simulink model "Constants"  (R2021a)
settings: Solver=FixedStepAuto  StartTime=0.0  StopTime=50  FixedStep=1e-3  RelTol=1e-3  EnableMultiTasking=on
undefined symbols (not defined in the file): D0, D1, D10, D11, D12, D13, D2, D3, D4, D5, D6, D7, D8, D9, magnitude, PTA0, PTA1, PTA2, PTB23, PTB9, PTC16, PTC17, PTC2, PTC3, PTC4, PTD0, PTD1, PTD2, PTD3
libraries: frdmk64flib x19, dspstat3 x1
settings Model: SimulationMode=external  PacingRate=0.250000  ExtModeTrigDuration=5  Creator=Arun Mistry  LastModifiedBy=Arun Mistry
settings OptimizationCC: EnhancedBackFolding=on  PassReuseOutputArgsAs=Individual arguments  ZeroExternalMemoryAtStartup=off  ZeroInternalMemoryAtStartup=off  MaxStackSize=64  OptimizeBlockOrder=speed  DifferentSizesBufferReuse=on  OptimizationCustomize=off  EfficientTunableParamExpr=on
settings DebuggingCC: ParameterTunabilityLossMsg=error
settings HardwareCC: ProdBitPerPointer=32  ProdBitPerSizeT=32  ProdBitPerPtrDiffT=32  ProdLargestAtomicInteger=Long  ProdLargestAtomicFloat=Double  ProdWordSize=32  ProdHWDeviceType=ARM Compatible->ARM Cortex
settings SFSimCC: MATLABDynamicMemAlloc=off
settings RTWCC: SystemTargetFile=ert.tlc  HardwareBoard=NXP FRDM-K64F  TLCOptions="-aInlineSetEventsForThisBaseRateFcn=TLC_FALSE -aSuppressMultiTaskScheduler=TLC_FALSE  -aRateBasedStepFcn=0"  TemplateMakefile=ert_default_tmf  Toolchain=GNU Tools for ARM Embedded Processors
settings CodeAppCC: ForceParamTrailComments=on  IgnoreCustomStorageClasses=off  OperatorAnnotations=on  SimulinkDataObjDesc=on  SFDataObjDesc=on  InsertBlockDesc=on
settings ERTTargetCC: ExtModeTransport=4  ExtModeMexFile=sendToCommService

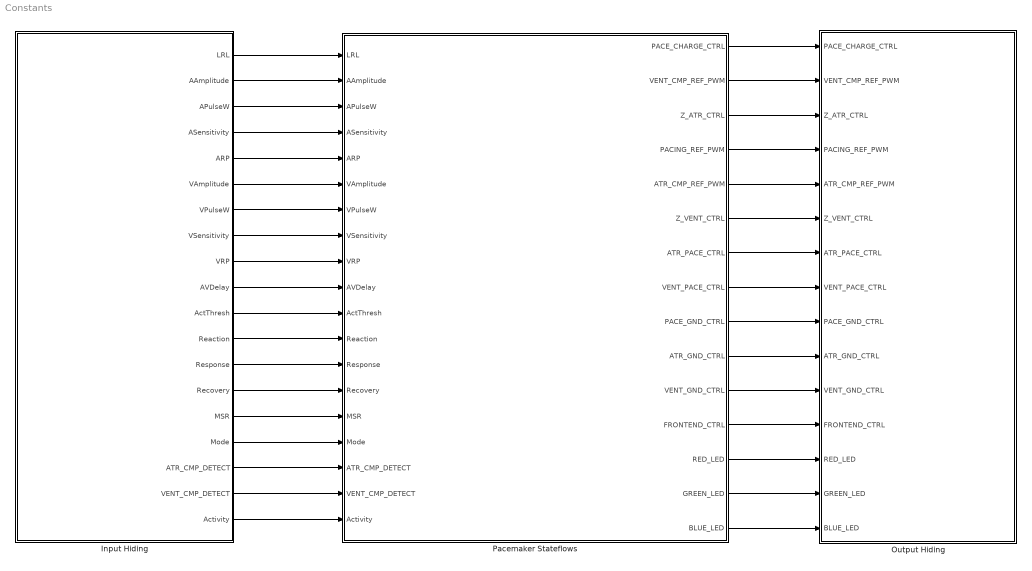
== system Constants ==
  Input Hiding : Subsystem
  Output Hiding : Subsystem
  Pacemaker Stateflows : Stateflow chart  TreatAsAtomicUnit=on
      settings: PortSchema="{\"entries\":[{\"content\":{\"sides\":[{\"content\":{\"connectorIds\":[\"In1\",\"In2\",\"In3\",\"In4\",\"In5\",\"In6\",\"In7\",\"In8\",\"In9\",\"In17\",\"In11\",\"In10\",\"In12\",\"In14\",\"In19\",\"In13\",\"In15\",\"In16\",\"In18\"]},\"type\":\"ConnectorPlacement.EquallySpacedRectSide\",\"uuid\":\"6f24296b-9994-4871-8227-e053a3629335\"},{\"content\":{\"connectorIds\":[\"Out1\",\"Out2\",\"Out3\",\"Out4\",\"Out5\",\"Out6\",\"Out7\",\"Out8\",\"Out9\",\"Out10\",\"Out11\",\"Out12\",\"Out13\",\"Out14\",\"Out15\"],\"side\":\"RIGHT\"},\"type\":\"ConnectorPlacement.EquallySpacedRectSide\",\"uuid\":\"36cf1f29-c3ea-48aa-b003-da737efff16a\"},{\"content\":{\"connectorIds\":[],\"side\":\"TOP\"},\"type\":\"ConnectorPlacement.EquallySpacedRectSide\",\"uuid\":\"8330eb51-0bc3-4d96-96ed-331fbb159cdb\"}]},\"type\":\"ConnectorPlacement.EquallySpacedConnector\",\"uuid\":\"1e79ed8a-065e-4a3c-97dd-23eb49490e0b\"}],\"packageUris\":[\"http://schema.mathworks.com/mf0/Connector/R2020b\"],\"version\":\"1.0\"}"
  wires:
  Pacemaker Stateflows/1(PACE_CHARGE_CTRL) -> Output Hiding/1(PACE_CHARGE_CTRL)
  Input Hiding/17(ATR_CMP_DETECT) -> Pacemaker Stateflows/15(ATR_CMP_DETECT)
  Input Hiding/7(VPulseW) -> Pacemaker Stateflows/7(VPulseW)
  Input Hiding/18(VENT_CMP_DETECT) -> Pacemaker Stateflows/16(VENT_CMP_DETECT)
  Pacemaker Stateflows/3(Z_ATR_CTRL) -> Output Hiding/3(Z_ATR_CTRL)
  Input Hiding/3(APulseW) -> Pacemaker Stateflows/3(APulseW)
  Pacemaker Stateflows/7(ATR_PACE_CTRL) -> Output Hiding/7(ATR_PACE_CTRL)
  Pacemaker Stateflows/10(ATR_GND_CTRL) -> Output Hiding/10(ATR_GND_CTRL)
  Input Hiding/16(Mode) -> Pacemaker Stateflows/13(Mode)
  Input Hiding/2(AAmplitude) -> Pacemaker Stateflows/2(AAmplitude)
  Input Hiding/6(VAmplitude) -> Pacemaker Stateflows/6(VAmplitude)
  Pacemaker Stateflows/6(Z_VENT_CTRL) -> Output Hiding/6(Z_VENT_CTRL)
  Pacemaker Stateflows/4(PACING_REF_PWM) -> Output Hiding/4(PACING_REF_PWM)
  Pacemaker Stateflows/11(VENT_GND_CTRL) -> Output Hiding/11(VENT_GND_CTRL)
  Pacemaker Stateflows/9(PACE_GND_CTRL) -> Output Hiding/9(PACE_GND_CTRL)
  Pacemaker Stateflows/8(VENT_PACE_CTRL) -> Output Hiding/8(VENT_PACE_CTRL)
  Input Hiding/1(LRL) -> Pacemaker Stateflows/1(LRL)
  Pacemaker Stateflows/15(BLUE_LED) -> Output Hiding/15(BLUE_LED)
  Input Hiding/4(ASensitivity) -> Pacemaker Stateflows/4(ASensitivity)
  Pacemaker Stateflows/12(FRONTEND_CTRL) -> Output Hiding/12(FRONTEND_CTRL)
  Input Hiding/9(VRP) -> Pacemaker Stateflows/9(VRP)
  Input Hiding/8(VSensitivity) -> Pacemaker Stateflows/8(VSensitivity)
  Input Hiding/5(ARP) -> Pacemaker Stateflows/5(ARP)
  Pacemaker Stateflows/14(GREEN_LED) -> Output Hiding/14(GREEN_LED)
  Pacemaker Stateflows/13(RED_LED) -> Output Hiding/13(RED_LED)
  Pacemaker Stateflows/5(ATR_CMP_REF_PWM) -> Output Hiding/5(ATR_CMP_REF_PWM)
  Pacemaker Stateflows/2(VENT_CMP_REF_PWM) -> Output Hiding/2(VENT_CMP_REF_PWM)
  Input Hiding/10(AVDelay) -> Pacemaker Stateflows/17(AVDelay)
  Input Hiding/19(Activity) -> Pacemaker Stateflows/18(Activity)
  Input Hiding/12(Reaction) -> Pacemaker Stateflows/10(Reaction)
  Input Hiding/13(Response) -> Pacemaker Stateflows/12(Response)
  Input Hiding/14(Recovery) -> Pacemaker Stateflows/14(Recovery)
  Input Hiding/15(MSR) -> Pacemaker Stateflows/19(MSR)
  Input Hiding/11(ActThresh) -> Pacemaker Stateflows/11(ActThresh)

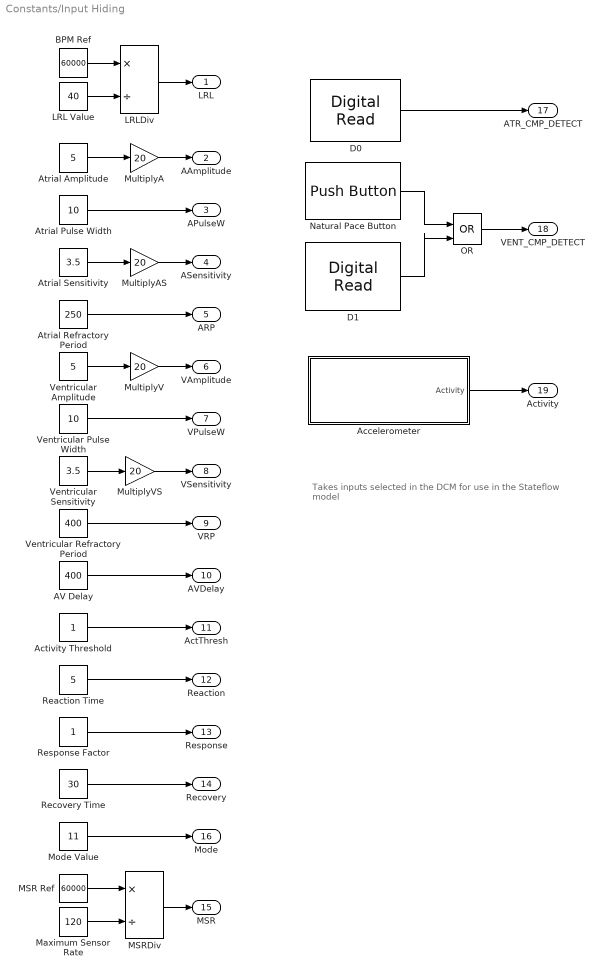
== system Constants/Input Hiding ==
  note: Takes inputs selected in the DCM for use in the Stateflow model
  AV Delay : Constant  Value=400  OutDataTypeStr=uint16
  Accelerometer : Subsystem
  Activity Threshold : Constant  OutDataTypeStr=double
  Atrial Amplitude : Constant  Value=5  OutDataTypeStr=double
  Atrial Pulse Width : Constant  Value=10  OutDataTypeStr=uint16
  Atrial Refractory Period : Constant  Value=250  OutDataTypeStr=uint16
  Atrial Sensitivity : Constant  Value=3.5  OutDataTypeStr=double
  BPM Ref : Constant  Value=60000  OutDataTypeStr=uint16
  D0 : frdmk64flib/Digital Read  Whichpin=PTC16 (D0)  SampleTime=-1
  D1 : frdmk64flib/Digital Read  Whichpin=PTC17 (D1)  SampleTime=-1
  LRL Value : Constant  Value=40  OutDataTypeStr=uint16
  LRLDiv : Product  Inputs=*/  OutDataTypeStr=uint16  RndMeth=Round
  MSR Ref : Constant  Value=60000  OutDataTypeStr=uint16
  MSRDiv : Product  Inputs=*/  OutDataTypeStr=uint16  RndMeth=Round
  Maximum Sensor Rate : Constant  Value=120  OutDataTypeStr=uint16
  Mode Value : Constant  Value=11  OutDataTypeStr=uint16
  MultiplyA : Gain  Gain=20  OutDataTypeStr=uint16
  MultiplyAS : Gain  Gain=20  OutDataTypeStr=uint16
  MultiplyV : Gain  Gain=20  OutDataTypeStr=uint16
  MultiplyVS : Gain  Gain=20  OutDataTypeStr=uint16
  Natural Pace Button : frdmk64flib/Push Button  Whichswitch=SW3  SampleTime1=-1
  OR : Logic  Operator=OR  IconShape=distinctive  AllPortsSameDT=off  OutDataTypeStr=boolean
  Reaction Time : Constant  Value=5  OutDataTypeStr=uint16
  Recovery Time : Constant  Value=30  OutDataTypeStr=uint16
  Response Factor : Constant  OutDataTypeStr=uint16
  Ventricular Amplitude : Constant  Value=5  OutDataTypeStr=double
  Ventricular Pulse Width : Constant  Value=10  OutDataTypeStr=uint16
  Ventricular Refractory Period : Constant  Value=400  OutDataTypeStr=uint16
  Ventricular Sensitivity : Constant  Value=3.5  OutDataTypeStr=double
  LRL : Outport  OutDataTypeStr=uint16
  AAmplitude : Outport  Port=2  OutDataTypeStr=uint16
  APulseW : Outport  Port=3  OutDataTypeStr=uint16
  ASensitivity : Outport  Port=4  OutDataTypeStr=uint16
  ARP : Outport  Port=5  OutDataTypeStr=uint16
  VAmplitude : Outport  Port=6  OutDataTypeStr=uint16
  VPulseW : Outport  Port=7  OutDataTypeStr=uint16
  VSensitivity : Outport  Port=8  OutDataTypeStr=uint16
  VRP : Outport  Port=9  OutDataTypeStr=uint16
  AVDelay : Outport  Port=10  OutDataTypeStr=uint16
  ActThresh : Outport  Port=11  OutDataTypeStr=double
  Reaction : Outport  Port=12  OutDataTypeStr=uint16
  Response : Outport  Port=13  OutDataTypeStr=uint16
  Recovery : Outport  Port=14  OutDataTypeStr=uint16
  MSR : Outport  Port=15  OutDataTypeStr=uint16
  Mode : Outport  Port=16  OutDataTypeStr=uint16
  ATR_CMP_DETECT : Outport  Port=17  OutDataTypeStr=boolean
  VENT_CMP_DETECT : Outport  Port=18  OutDataTypeStr=boolean
  Activity : Outport  Port=19  OutDataTypeStr=double
  wires:
  MultiplyAS/1 -> ASensitivity/1
  MultiplyVS/1 -> VSensitivity/1
  MultiplyA/1 -> AAmplitude/1
  LRLDiv/1 -> LRL/1
  Maximum Sensor Rate/1 -> MSRDiv/2
  Response Factor/1 -> Response/1
  Reaction Time/1 -> Reaction/1
  Natural Pace Button/1 -> OR/1
  OR/1 -> VENT_CMP_DETECT/1
  Mode Value/1 -> Mode/1
  Atrial Sensitivity/1 -> MultiplyAS/1
  Activity Threshold/1 -> ActThresh/1
  D1/1 -> OR/2
  Ventricular Refractory Period/1 -> VRP/1
  MSR Ref/1 -> MSRDiv/1
  MSRDiv/1 -> MSR/1
  Recovery Time/1 -> Recovery/1
  Accelerometer/1(Activity) -> Activity/1
  AV Delay/1 -> AVDelay/1
  Ventricular Sensitivity/1 -> MultiplyVS/1
  Ventricular Pulse Width/1 -> VPulseW/1
  LRL Value/1 -> LRLDiv/2
  BPM Ref/1 -> LRLDiv/1
  Atrial Refractory Period/1 -> ARP/1
  Ventricular Amplitude/1 -> MultiplyV/1
  MultiplyV/1 -> VAmplitude/1
  D0/1 -> ATR_CMP_DETECT/1
  Atrial Pulse Width/1 -> APulseW/1
  Atrial Amplitude/1 -> MultiplyA/1

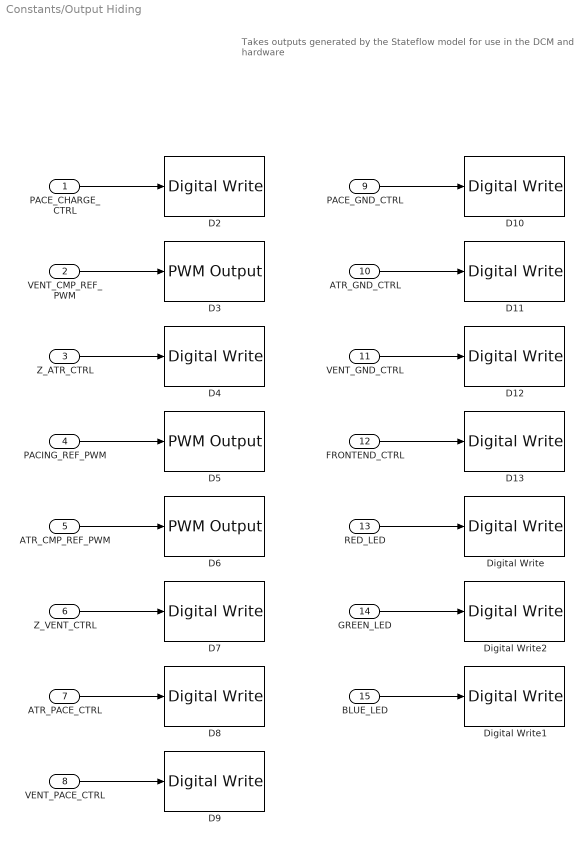
== system Constants/Output Hiding ==
  note: Takes outputs generated by the Stateflow model for use in the DCM and hardware
  PACE_CHARGE_CTRL : Inport  OutDataTypeStr=uint16
  VENT_CMP_REF_PWM : Inport  Port=2  OutDataTypeStr=uint16
  Z_ATR_CTRL : Inport  Port=3  OutDataTypeStr=uint16
  PACING_REF_PWM : Inport  Port=4  OutDataTypeStr=uint16
  ATR_CMP_REF_PWM : Inport  Port=5  OutDataTypeStr=uint16
  Z_VENT_CTRL : Inport  Port=6  OutDataTypeStr=uint16
  ATR_PACE_CTRL : Inport  Port=7  OutDataTypeStr=uint16
  VENT_PACE_CTRL : Inport  Port=8  OutDataTypeStr=uint16
  PACE_GND_CTRL : Inport  Port=9  OutDataTypeStr=uint16
  ATR_GND_CTRL : Inport  Port=10  OutDataTypeStr=uint16
  VENT_GND_CTRL : Inport  Port=11  OutDataTypeStr=uint16
  FRONTEND_CTRL : Inport  Port=12  OutDataTypeStr=uint16
  RED_LED : Inport  Port=13  OutDataTypeStr=uint16
  GREEN_LED : Inport  Port=14  OutDataTypeStr=uint16
  BLUE_LED : Inport  Port=15  OutDataTypeStr=uint16
  D10 : frdmk64flib/Digital Write  Whichpin=PTD0 (D10)
  D11 : frdmk64flib/Digital Write  Whichpin=PTD2 (D11)
  D12 : frdmk64flib/Digital Write  Whichpin=PTD3 (D12)
  D13 : frdmk64flib/Digital Write  Whichpin=PTD1 (D13)
  D2 : frdmk64flib/Digital Write  Whichpin=PTB9 (D2)
  D3 : frdmk64flib/PWM Output  Whichpin=PTA1 (D3)  InitialFrequency=2000  InitialDutyCycle=100
  D4 : frdmk64flib/Digital Write  Whichpin=PTB23 (D4)
  D5 : frdmk64flib/PWM Output  Whichpin=PTA2 (D5)  InitialFrequency=2000  InitialDutyCycle=100
  D6 : frdmk64flib/PWM Output  Whichpin=PTC2 (D6)  InitialFrequency=2000  InitialDutyCycle=100
  D7 : frdmk64flib/Digital Write  Whichpin=PTC3 (D7)
  "D8 " : frdmk64flib/Digital Write  Whichpin=PTA0 (D8)
  D9 : frdmk64flib/Digital Write  Whichpin=PTC4 (D9)
  Digital Write : frdmk64flib/Digital Write  Whichpin=RED_LED
  Digital Write1 : frdmk64flib/Digital Write  Whichpin=BLUE_LED
  Digital Write2 : frdmk64flib/Digital Write  Whichpin=GREEN_LED
  wires:
  VENT_PACE_CTRL/1 -> D9/1
  ATR_CMP_REF_PWM/1 -> D6/1
  PACE_GND_CTRL/1 -> D10/1
  VENT_CMP_REF_PWM/1 -> D3/1
  PACING_REF_PWM/1 -> D5/1
  ATR_GND_CTRL/1 -> D11/1
  ATR_PACE_CTRL/1 -> "D8 "/1
  PACE_CHARGE_CTRL/1 -> D2/1
  FRONTEND_CTRL/1 -> D13/1
  VENT_GND_CTRL/1 -> D12/1
  Z_ATR_CTRL/1 -> D4/1
  Z_VENT_CTRL/1 -> D7/1
  RED_LED/1 -> Digital Write/1
  BLUE_LED/1 -> Digital Write1/1
  GREEN_LED/1 -> Digital Write2/1

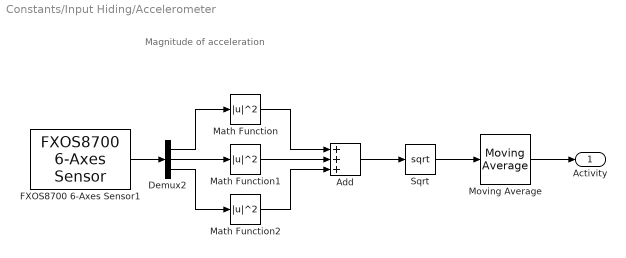
== system Constants/Input Hiding/Accelerometer ==
  note: Magnitude of acceleration
  Add : Sum  Inputs=+++
  Demux2 : Demux  Outputs=3
  FXOS8700 6-Axes Sensor1 : frdmk64flib/FXOS8700 6-Axes Sensor  Activesensor=Accelerometer only  ODR=100Hz  HybridODR=400Hz  Accelfullrange=-8g to +8g  SampleTime=1/100
  Math Function : Math  Operator=magnitude^2  SignedPower=on  OutDataTypeStr=double  SaturateOnIntegerOverflow=on
  Math Function1 : Math  Operator=magnitude^2  SignedPower=on  OutDataTypeStr=double  SaturateOnIntegerOverflow=on
  Math Function2 : Math  Operator=magnitude^2  SignedPower=on  OutDataTypeStr=double  SaturateOnIntegerOverflow=on
  Moving Average : dspstat3/Moving Average  Method=Sliding window  ForgettingFactorPort=off  SpecifyWindowLength=on  WindowLength=30  ForgettingFactor=0.9  SimulateUsing=Code generation
  Sqrt : Sqrt  SaturateOnIntegerOverflow=on
  Activity : Outport  OutDataTypeStr=double  SourceOfInitialOutputValue=Input signal
  wires:
  Sqrt/1 -> Moving Average/1
  FXOS8700 6-Axes Sensor1/1 -> Demux2/1
  Math Function/1 -> Add/1
  Add/1 -> Sqrt/1
  Math Function2/1 -> Add/3
  Demux2/2 -> Math Function1/1
  Math Function1/1 -> Add/2
  Demux2/1 -> Math Function/1
  Demux2/3 -> Math Function2/1
  Moving Average/1 -> Activity/1

== stateflow chart Constants/Pacemaker Stateflows ==
  note: Mode selected from DCM changes which State will be run
  state AOO
    entry:
    VENT_PACE_CTRL = 0; VENT_GND_CTRL = 0; PACE_GND_CTRL = 1;
    Z_VENT_CTRL = 0; Z_ATR_CTRL = 0;
    during: PACING_REF_PWM = AAmplitude;
    note: Duration of Pulse
    state PACE_ATR
      entry:
      PACE_CHARGE_CTRL = 0;
      ATR_GND_CTRL = 0;
      ATR_PACE_CTRL = 1;
      RED_LED = 1;
    state C22_CHARGE
      entry:
      PACE_CHARGE_CTRL = 1;
      ATR_PACE_CTRL = 0;
      ATR_GND_CTRL = 1;
      RED_LED = 0;
    note: Wait for LRL before Pulse
    note: Toggle values between
        | C22_CHARGE and PACE_ATR
    (default) -> AOO.C22_CHARGE
    AOO.PACE_ATR -> AOO.C22_CHARGE : after(APulseW,msec)
    AOO.C22_CHARGE -> AOO.PACE_ATR : after(LRL-APulseW,msec)
  state MODE_SELECTION
    entry:
    GREEN_LED = 0;
    RED_LED = 0;
    BLUE_LED = 0;
    FRONTEND_CTRL = 0;
    PACING_REF_PWM = 0;
    ATR_CMP_REF_PWM = 0;
    VENT_CMP_REF_PWM = 0;
    PACE_CHARGE_CTRL= 0;
    PACE_GND_CTRL= 0;
    ATR_PACE_CTRL = 0;
    ATR_GND_CTRL = 0;
    VENT_PACE_CTRL = 0;
    VENT_GND_CTRL = 0;
    Z_ATR_CTRL = 0;
    Z_VENT_CTRL = 0;
    note: Reset the values above
        | upon switching modes
  state VOO
    entry:
    ATR_PACE_CTRL = 0; ATR_GND_CTRL = 0; PACE_GND_CTRL = 1;
    Z_ATR_CTRL = 0; Z_VENT_CTRL = 0;
    during: PACING_REF_PWM = VAmplitude;
    note: Duration of high
    state PACE_VENT
      entry:
      PACE_CHARGE_CTRL = 0;
      VENT_GND_CTRL = 0;
      VENT_PACE_CTRL = 1;
      BLUE_LED = 1;
    state C22_CHARGE
      entry:
      VENT_PACE_CTRL = 0;
      VENT_GND_CTRL = 1;
      PACE_CHARGE_CTRL = 1;
      BLUE_LED = 0;
    note: Duration of low
    note: Toggle values between
        | C22_CHARGE and PACE_VENT
    (default) -> VOO.C22_CHARGE
    VOO.PACE_VENT -> VOO.C22_CHARGE : after(VPulseW,msec)
    VOO.C22_CHARGE -> VOO.PACE_VENT : after(LRL-VPulseW,msec)
  note: Mode 1
  note: Mode 2
  state AAI
    entry: VENT_PACE_CTRL = 0; VENT_GND_CTRL = 0; PACE_GND_CTRL = 1;
    Z_VENT_CTRL = 0; Z_ATR_CTRL = 0; FRONTEND_CTRL = 1;
    during: PACING_REF_PWM = AAmplitude; ATR_CMP_REF_PWM=ASensitivity;
    state PACE_ATR
      entry:
      ATR_PACE_CTRL = 1;
      PACE_CHARGE_CTRL = 0;
      ATR_GND_CTRL = 0;
      RED_LED = 1;
    state C22_CHARGE
      entry:
      ATR_PACE_CTRL = 0;
      PACE_CHARGE_CTRL = 1;
      ATR_GND_CTRL = 1;
    state REFRACTORY
      entry: RED_LED = 0; PACE_CHARGE_CTRL = 1;
      ATR_PACE_CTRL = 0;  ATR_GND_CTRL = 1;
      exit: GREEN_LED = 0;
    (default) -> AAI.C22_CHARGE
    AAI.C22_CHARGE -> AAI.PACE_ATR [order 2] : after(LRL - ARP, msec)
    AAI.C22_CHARGE -> AAI.REFRACTORY [order 1] : after(APulseW,msec)
        | [ATR_CMP_DETECT]
        | { GREEN_LED = 1; }
    AAI.REFRACTORY -> AAI.C22_CHARGE : after(ARP, msec)
    AAI.PACE_ATR -> AAI.REFRACTORY : after(APulseW, msec)
  state VVI
    entry: ATR_PACE_CTRL = 0; ATR_GND_CTRL = 0; PACE_GND_CTRL = 1;
    Z_VENT_CTRL = 0; Z_ATR_CTRL = 0; FRONTEND_CTRL = 1;
    during: PACING_REF_PWM = VAmplitude; VENT_CMP_REF_PWM = VSensitivity;
    state PACE_VENT
      entry:
      PACE_CHARGE_CTRL = 0;
      VENT_PACE_CTRL = 1;
      VENT_GND_CTRL = 0;
      RED_LED = 1;
    state C22_CHARGE
      entry:
      PACE_CHARGE_CTRL = 1;
      VENT_PACE_CTRL = 0;
      VENT_GND_CTRL = 1;
    state REFRACTORY
      entry: RED_LED = 0; PACE_CHARGE_CTRL = 1;
      VENT_PACE_CTRL = 0;  VENT_GND_CTRL = 1;
      exit: GREEN_LED = 0;
    (default) -> VVI.C22_CHARGE
    VVI.C22_CHARGE -> VVI.PACE_VENT [order 2] : after(LRL - VRP, msec)
    VVI.C22_CHARGE -> VVI.REFRACTORY [order 1] : after(VPulseW,msec)
        | [VENT_CMP_DETECT]
        | { GREEN_LED = 1; }
    VVI.REFRACTORY -> VVI.C22_CHARGE : after(VRP, msec)
    VVI.PACE_VENT -> VVI.REFRACTORY : after(VPulseW, msec)
  note: Mode 3
  note: Mode 4
  state AOOR
    entry:
    Z_VENT_CTRL = 0;
    Z_ATR_CTRL = 0;
    VENT_PACE_CTRL = 0;
    VENT_GND_CTRL = 0;
    PACE_GND_CTRL = 1;
    during:
    PACING_REF_PWM = AAmplitude;
    state PACE [parallel]
      settings: executionOrder=1
      state PACE_ATR
        entry:
        PACE_CHARGE_CTRL = 0;
        ATR_GND_CTRL = 0;
        ATR_PACE_CTRL = 1;
        RED_LED = 1;
      state C22_CHARGE
        entry:
        PACE_CHARGE_CTRL = 1;
        ATR_PACE_CTRL = 0;
        ATR_GND_CTRL = 1;
        RED_LED = 0;
      (default) -> AOOR.PACE.C22_CHARGE
      AOOR.PACE.PACE_ATR -> AOOR.PACE.C22_CHARGE : after(APulseW,msec)
      AOOR.PACE.C22_CHARGE -> AOOR.PACE.PACE_ATR : after(ceil(ModRate)-APulseW,msec)
    state MODULATION [parallel]
      during: increment = double(LRL-MSR)/double(Reaction); decrement = double(LRL - MSR)/double(Recovery);
      Target = double(LRL) - (Activity - ActThresh)/double(17 - Response)*2000;
      settings: executionOrder=2
      state STEPUP
        entry:
        ModRate = ModRate - increment/100;
      state START
        entry:
        ModRate = double(LRL);
      state MAXIMUM
        entry:
        ModRate = double(MSR);
      state STEPDOWN
        entry:
        ModRate = ModRate + decrement/100;
      AOOR.MODULATION.STEPUP -> AOOR.MODULATION.STEPUP [order 2] : after(10,msec)[ModRate > Target]
      AOOR.MODULATION.START -> AOOR.MODULATION.STEPUP : [Target < LRL]
      AOOR.MODULATION.STEPUP -> AOOR.MODULATION.MAXIMUM [order 1] : [ModRate <= MSR]
      AOOR.MODULATION.STEPUP -> AOOR.MODULATION.STEPDOWN [order 3] : after(10,msec)
          | [ModRate <= Target]
      AOOR.MODULATION.STEPDOWN -> AOOR.MODULATION.STEPUP [order 3] : after(10,msec)
          | [ModRate >= Target]
      (default) -> AOOR.MODULATION.START
      AOOR.MODULATION.STEPDOWN -> AOOR.MODULATION.START [order 1] : [ModRate >= LRL]
      AOOR.MODULATION.MAXIMUM -> AOOR.MODULATION.STEPDOWN : [Target > MSR]
      AOOR.MODULATION.STEPDOWN -> AOOR.MODULATION.STEPDOWN [order 2] : after(10, msec)[ModRate < Target]
  state VOOR
    entry:
    ATR_PACE_CTRL = 0;
    ATR_GND_CTRL = 0;
    PACE_GND_CTRL = 1;
    Z_ATR_CTRL = 0;
    Z_VENT_CTRL = 0;
    during:
    PACING_REF_PWM = VAmplitude;
    state PACE [parallel]
      settings: executionOrder=1
      state PACE_VENT
        entry:
        PACE_CHARGE_CTRL = 0;
        VENT_GND_CTRL = 0;
        VENT_PACE_CTRL = 1;
        BLUE_LED = 1;
      state C22_CHARGE
        entry:
        VENT_PACE_CTRL = 0;
        VENT_GND_CTRL = 1;
        PACE_CHARGE_CTRL = 1;
        BLUE_LED = 0;
      (default) -> VOOR.PACE.C22_CHARGE
      VOOR.PACE.PACE_VENT -> VOOR.PACE.C22_CHARGE : after(VPulseW,msec)
      VOOR.PACE.C22_CHARGE -> VOOR.PACE.PACE_VENT : after(ceil(ModRate)-VPulseW,msec)
    state MODULATION [parallel]
      during: increment = double(LRL-MSR)/double(Reaction); decrement = double(LRL - MSR)/double(Recovery);
      Target = double(LRL) - (Activity - ActThresh)/double(17 - Response)*2000;
      settings: executionOrder=2
      state RATEUP
        entry:
        ModRate = ModRate - increment/100;
      state MINIMUM
        entry:
        ModRate = double(LRL);
      state MAXIMUM
        entry:
        ModRate = double(MSR);
      state RATEDOWN
        entry:
        ModRate = ModRate + decrement/100;
      RATEUP -> RATEUP [order 2] : after(10,msec)[ModRate > Target]
      MINIMUM -> RATEUP : [Target < LRL]
      RATEUP -> VOOR.MODULATION.MAXIMUM [order 1] : [ModRate <= MSR]
      RATEUP -> RATEDOWN [order 3] : after(10,msec)
          | [ModRate <= Target]
      RATEDOWN -> RATEUP [order 3] : after(10,msec)
          | [ModRate >= Target]
      (default) -> MINIMUM
      RATEDOWN -> MINIMUM [order 1] : [ModRate >= LRL]
      VOOR.MODULATION.MAXIMUM -> RATEDOWN : [Target > MSR]
      RATEDOWN -> RATEDOWN [order 2] : after(10, msec)[ModRate < Target]
  note: Mode 5
  note: Mode 6
  state AAIR
    entry: VENT_PACE_CTRL = 0; VENT_GND_CTRL = 0;  PACE_GND_CTRL = 1;
    Z_VENT_CTRL = 0; Z_ATR_CTRL = 0; FRONTEND_CTRL = 1;
    during: PACING_REF_PWM = AAmplitude; ATR_CMP_REF_PWM=ASensitivity;
    state PACE [parallel]
      settings: executionOrder=1
      state PACE_ATR
        entry:
        ATR_PACE_CTRL = 1;
        PACE_CHARGE_CTRL = 0;
        ATR_GND_CTRL = 0;
        RED_LED = 1;
      state C22_CHARGE
        entry:
        ATR_PACE_CTRL = 0;
        PACE_CHARGE_CTRL = 1;
        ATR_GND_CTRL = 1;
      state REFRACTORY
        entry: RED_LED = 0; PACE_CHARGE_CTRL = 1;
        ATR_PACE_CTRL = 0;  ATR_GND_CTRL = 1;
        exit: GREEN_LED = 0;
      (default) -> AAIR.PACE.C22_CHARGE
      AAIR.PACE.C22_CHARGE -> AAIR.PACE.PACE_ATR [order 2] : after(ceil(ModRate) - ARP, msec)
      AAIR.PACE.C22_CHARGE -> AAIR.PACE.REFRACTORY [order 1] : after(APulseW,msec)
          | [ATR_CMP_DETECT]
          | { GREEN_LED = 1; }
      AAIR.PACE.REFRACTORY -> AAIR.PACE.C22_CHARGE : after(ARP, msec)
      AAIR.PACE.PACE_ATR -> AAIR.PACE.REFRACTORY : after(APulseW, msec)
    state MODULATION [parallel]
      during: increment = double(LRL-MSR)/double(Reaction); decrement = double(LRL - MSR)/double(Recovery);
      Target = double(LRL) - (Activity - ActThresh)/double(17 - Response)*2000;
      settings: executionOrder=2
      state STEPUP
        entry:
        ModRate = ModRate - increment/100;
      state START
        entry:
        ModRate = double(LRL);
      state MAXIMUM
        entry:
        ModRate = double(MSR);
      state STEPDOWN
        entry:
        ModRate = ModRate + decrement/100;
      AAIR.MODULATION.STEPUP -> AAIR.MODULATION.STEPUP [order 2] : after(10,msec)[ModRate > Target]
      AAIR.MODULATION.START -> AAIR.MODULATION.STEPUP : [Target < LRL]
      AAIR.MODULATION.STEPUP -> AAIR.MODULATION.MAXIMUM [order 1] : [ModRate <= MSR]
      AAIR.MODULATION.STEPUP -> AAIR.MODULATION.STEPDOWN [order 3] : after(10,msec)
          | [ModRate <= Target]
      AAIR.MODULATION.STEPDOWN -> AAIR.MODULATION.STEPUP [order 3] : after(10,msec)
          | [ModRate >= Target]
      (default) -> AAIR.MODULATION.START
      AAIR.MODULATION.STEPDOWN -> AAIR.MODULATION.START [order 1] : [ModRate >= LRL]
      AAIR.MODULATION.MAXIMUM -> AAIR.MODULATION.STEPDOWN : [Target > MSR]
      AAIR.MODULATION.STEPDOWN -> AAIR.MODULATION.STEPDOWN [order 2] : after(10, msec)[ModRate < Target]
  state VVIR
    entry: ATR_PACE_CTRL = 0; ATR_GND_CTRL = 0; PACE_GND_CTRL = 1;
    Z_VENT_CTRL = 0; Z_ATR_CTRL = 0; FRONTEND_CTRL = 1;
    during:  PACING_REF_PWM = VAmplitude; VENT_CMP_REF_PWM = VSensitivity;
    state PACE [parallel]
      settings: executionOrder=1
      state PACE_VENT
        entry:
        PACE_CHARGE_CTRL = 0;
        VENT_PACE_CTRL = 1;
        VENT_GND_CTRL = 0;
        RED_LED = 1;
      state C22_CHARGE
        entry:
        PACE_CHARGE_CTRL = 1;
        VENT_PACE_CTRL = 0;
        VENT_GND_CTRL = 1;
      state REFRACTORY
        entry: RED_LED = 0; PACE_CHARGE_CTRL = 1;
        VENT_PACE_CTRL = 0;  VENT_GND_CTRL = 1;
        exit: GREEN_LED = 0;
      VVIR.PACE.C22_CHARGE -> VVIR.PACE.PACE_VENT [order 2] : after(ceil(ModRate) - VRP, msec)
      (default) -> VVIR.PACE.C22_CHARGE
      VVIR.PACE.C22_CHARGE -> VVIR.PACE.REFRACTORY [order 1] : after(VPulseW,msec)
          | [VENT_CMP_DETECT]
          | { GREEN_LED = 1; }
      VVIR.PACE.REFRACTORY -> VVIR.PACE.C22_CHARGE : after(VRP, msec)
      VVIR.PACE.PACE_VENT -> VVIR.PACE.REFRACTORY : after(VPulseW, msec)
    state MODULATION [parallel]
      during: increment = double(LRL-MSR)/double(Reaction); decrement = double(LRL - MSR)/double(Recovery);
      Target = double(LRL) - (Activity - ActThresh)/double(17 - Response)*2000;
      settings: executionOrder=2
      state STEPUP
        entry:
        ModRate = ModRate - increment/100;
      state START
        entry:
        ModRate = double(LRL);
      state MAXIMUM
        entry:
        ModRate = double(MSR);
      state STEPDOWN
        entry:
        ModRate = ModRate + decrement/100;
      VVIR.MODULATION.STEPUP -> VVIR.MODULATION.STEPUP [order 2] : after(10,msec)[ModRate > Target]
      VVIR.MODULATION.START -> VVIR.MODULATION.STEPUP : [Target < LRL]
      VVIR.MODULATION.STEPUP -> VVIR.MODULATION.MAXIMUM [order 1] : [ModRate <= MSR]
      VVIR.MODULATION.STEPUP -> VVIR.MODULATION.STEPDOWN [order 3] : after(10,msec)
          | [ModRate <= Target]
      VVIR.MODULATION.STEPDOWN -> VVIR.MODULATION.STEPUP [order 3] : after(10,msec)
          | [ModRate >= Target]
      (default) -> VVIR.MODULATION.START
      VVIR.MODULATION.STEPDOWN -> VVIR.MODULATION.START [order 1] : [ModRate >= LRL]
      VVIR.MODULATION.MAXIMUM -> VVIR.MODULATION.STEPDOWN : [Target > MSR]
      VVIR.MODULATION.STEPDOWN -> VVIR.MODULATION.STEPDOWN [order 2] : after(10, msec)[ModRate < Target]
  note: Mode 7
  note: Mode 8
  state DOO
    entry: Z_VENT_CTRL = 0; Z_ATR_CTRL = 0; PACE_GND_CTRL = 1;
    note: Both low,
        | prep for ATR pulse
    note: Pace ATR
    state PACE_ATR
      entry:
      PACE_CHARGE_CTRL = 0;
      ATR_GND_CTRL = 0;
      VENT_GND_CTRL = 0;
      ATR_PACE_CTRL = 1;
      RED_LED = 1;
    state C22_CHARGE
      entry:
      ATR_PACE_CTRL = 0;
      VENT_PACE_CTRL = 0;
      PACING_REF_PWM = AAmplitude;
      PACE_CHARGE_CTRL = 1;
      ATR_GND_CTRL = 0;
      VENT_GND_CTRL = 1;
      BLUE_LED = 0;
    note: Duration of ATR pulse high
    note: Duration of VENT pulse high
    state AVDelay_PERIOD
      entry:
      ATR_PACE_CTRL = 0;
      VENT_PACE_CTRL = 0;
      PACING_REF_PWM = VAmplitude;
      PACE_CHARGE_CTRL = 1;
      ATR_GND_CTRL = 1;
      VENT_GND_CTRL = 0;
      RED_LED = 0;
    state PACE_VENT
      entry:
      PACE_CHARGE_CTRL = 0;
      ATR_GND_CTRL = 0;
      VENT_GND_CTRL = 0;
      VENT_PACE_CTRL = 1;
      BLUE_LED = 1;
    note: Pace vent
    note: Both low, prep for VENT pulse
    (default) -> DOO.C22_CHARGE
    DOO.C22_CHARGE -> DOO.PACE_ATR : after(LRL-AVDelay-VPulseW,msec)
    DOO.PACE_ATR -> DOO.AVDelay_PERIOD : after(APulseW,msec)
    DOO.PACE_VENT -> DOO.C22_CHARGE : after(VPulseW, msec)
    DOO.AVDelay_PERIOD -> DOO.PACE_VENT : after(AVDelay-APulseW,msec)
  state DOOR
    entry: Z_VENT_CTRL = 0; Z_ATR_CTRL = 0; PACE_GND_CTRL = 1;
    state Pace [parallel]
      settings: executionOrder=1
      note: Both low,
          | prep for ATR pulse
      note: Pace ATR
      state PACE_ATR
        entry:
        PACE_CHARGE_CTRL = 0;
        ATR_GND_CTRL = 0;
        VENT_GND_CTRL = 0;
        ATR_PACE_CTRL = 1;
        RED_LED = 1;
      state C22_CHARGE
        entry:
        ATR_PACE_CTRL = 0;
        VENT_PACE_CTRL = 0;
        PACING_REF_PWM = AAmplitude;
        PACE_CHARGE_CTRL = 1;
        ATR_GND_CTRL = 0;
        VENT_GND_CTRL = 1;
        BLUE_LED = 0;
      note: Duration of ATR pulse high
      note: Duration of VENT pulse high
      state AVDelay_PERIOD
        entry:
        ATR_PACE_CTRL = 0;
        VENT_PACE_CTRL = 0;
        PACING_REF_PWM = VAmplitude;
        PACE_CHARGE_CTRL = 1;
        ATR_GND_CTRL = 1;
        VENT_GND_CTRL = 0;
        RED_LED = 0;
      state PACE_VENT
        entry:
        PACE_CHARGE_CTRL = 0;
        ATR_GND_CTRL = 0;
        VENT_GND_CTRL = 0;
        VENT_PACE_CTRL = 1;
        BLUE_LED = 1;
      note: Both low, prep for VENT pulse
      note: Pace vent
      (default) -> DOOR.Pace.C22_CHARGE
      DOOR.Pace.C22_CHARGE -> DOOR.Pace.PACE_ATR : after(ceil(ModRate)-AVDelay-VPulseW,msec)
      DOOR.Pace.PACE_ATR -> DOOR.Pace.AVDelay_PERIOD : after(APulseW,msec)
      DOOR.Pace.PACE_VENT -> DOOR.Pace.C22_CHARGE : after(VPulseW, msec)
      DOOR.Pace.AVDelay_PERIOD -> DOOR.Pace.PACE_VENT : after(AVDelay-APulseW,msec)
    state MODULATION [parallel]
      during: increment = double(LRL-MSR)/double(Reaction); decrement = double(LRL - MSR)/double(Recovery);
      Target = double(LRL) - (Activity - ActThresh)/double(17 - Response)*2000;
      settings: executionOrder=2
      state STEPUP
        entry:
        ModRate = ModRate - increment/100;
      state START
        entry:
        ModRate = double(LRL);
      state MAXIMUM
        entry:
        ModRate = double(MSR);
      state STEPDOWN
        entry:
        ModRate = ModRate + decrement/100;
      DOOR.MODULATION.STEPUP -> DOOR.MODULATION.STEPUP [order 2] : after(10,msec)[ModRate > Target]
      DOOR.MODULATION.START -> DOOR.MODULATION.STEPUP : [Target < LRL]
      DOOR.MODULATION.STEPUP -> DOOR.MODULATION.MAXIMUM [order 1] : [ModRate <= MSR]
      DOOR.MODULATION.STEPUP -> DOOR.MODULATION.STEPDOWN [order 3] : after(10,msec)
          | [ModRate <= Target]
      DOOR.MODULATION.STEPDOWN -> DOOR.MODULATION.STEPUP [order 3] : after(10,msec)
          | [ModRate >= Target]
      (default) -> DOOR.MODULATION.START
      DOOR.MODULATION.STEPDOWN -> DOOR.MODULATION.START [order 1] : [ModRate >= LRL]
      DOOR.MODULATION.MAXIMUM -> DOOR.MODULATION.STEPDOWN : [Target > MSR]
      DOOR.MODULATION.STEPDOWN -> DOOR.MODULATION.STEPDOWN [order 2] : after(10, msec)[ModRate < Target]
  state DDD
    entry: Z_VENT_CTRL = 0; Z_ATR_CTRL = 0; PACE_GND_CTRL = 1;
    during: ATR_CMP_REF_PWM = ASensitivity; VENT_CMP_REF_PWM = VSensitivity;
    state PACE_ATR
      entry:
      PACE_CHARGE_CTRL = 0;
      ATR_GND_CTRL = 0;
      VENT_GND_CTRL = 0;
      ATR_PACE_CTRL = 1;
      RED_LED = 1;
    state C22_CHARGE
      entry:
      ATR_PACE_CTRL = 0;
      VENT_PACE_CTRL = 0;
      PACING_REF_PWM = AAmplitude;
      PACE_CHARGE_CTRL = 1;
      ATR_GND_CTRL = 0;
      VENT_GND_CTRL = 1;
      BLUE_LED = 0;
      GREEN_LED = 0;
    state AVDelay_PERIOD
      entry:
      ATR_PACE_CTRL = 0;
      VENT_PACE_CTRL = 0;
      PACING_REF_PWM = VAmplitude;
      PACE_CHARGE_CTRL = 1;
      ATR_GND_CTRL = 1;
      VENT_GND_CTRL = 0;
      RED_LED = 0;
    state PACE_VENT
      entry:
      PACE_CHARGE_CTRL = 0;
      ATR_GND_CTRL = 0;
      VENT_GND_CTRL = 0;
      VENT_PACE_CTRL = 1;
      BLUE_LED = 1;
    (default) -> DDD.C22_CHARGE
    DDD.C22_CHARGE -> DDD.PACE_ATR [order 2] : after(LRL-AVDelay-VPulseW,msec)
    DDD.PACE_ATR -> DDD.AVDelay_PERIOD : after(APulseW,msec)
    DDD.C22_CHARGE -> DDD.AVDelay_PERIOD [order 1] : after(APulseW,msec)
        | [ATR_CMP_DETECT]
        | {GREEN_LED = 0;}
    DDD.AVDelay_PERIOD -> DDD.C22_CHARGE [order 1] : after(APulseW,msec)
        | [VENT_CMP_DETECT]
        | {GREEN_LED = 1;}
    DDD.PACE_VENT -> DDD.C22_CHARGE : after(VPulseW,msec)
    DDD.AVDelay_PERIOD -> DDD.PACE_VENT [order 2] : after(AVDelay-APulseW,msec)
  state DDDR
    entry: Z_VENT_CTRL = 0; Z_ATR_CTRL = 0; PACE_GND_CTRL = 1;
    during: ATR_CMP_REF_PWM=ASensitivity; VENT_CMP_REF_PWM = VSensitivity;
    state Pace [parallel]
      settings: executionOrder=1
      state PACE_ATR
        entry:
        PACE_CHARGE_CTRL = 0;
        ATR_GND_CTRL = 0;
        VENT_GND_CTRL = 0;
        ATR_PACE_CTRL = 1;
        RED_LED = 1;
      state C22_CHARGE
        entry:
        ATR_PACE_CTRL = 0;
        VENT_PACE_CTRL = 0;
        PACING_REF_PWM = AAmplitude;
        PACE_CHARGE_CTRL = 1;
        ATR_GND_CTRL = 0;
        VENT_GND_CTRL = 1;
        BLUE_LED = 0;
      state AVDelay_PERIOD
        entry:
        ATR_PACE_CTRL = 0;
        VENT_PACE_CTRL = 0;
        PACING_REF_PWM = VAmplitude;
        PACE_CHARGE_CTRL = 1;
        ATR_GND_CTRL = 1;
        VENT_GND_CTRL = 0;
        RED_LED = 0;
      state PACE_VENT
        entry:
        PACE_CHARGE_CTRL = 0;
        ATR_GND_CTRL = 0;
        VENT_GND_CTRL = 0;
        VENT_PACE_CTRL = 1;
        BLUE_LED = 1;
      (default) -> DDDR.Pace.C22_CHARGE
      DDDR.Pace.C22_CHARGE -> DDDR.Pace.PACE_ATR [order 2] : after(ceil(ModRate)-AVDelay-VPulseW,msec)
      DDDR.Pace.C22_CHARGE -> DDDR.Pace.AVDelay_PERIOD [order 1] : after(APulseW,msec)
          | [ATR_CMP_DETECT]
      DDDR.Pace.PACE_ATR -> DDDR.Pace.AVDelay_PERIOD : after(APulseW,msec)
      DDDR.Pace.AVDelay_PERIOD -> DDDR.Pace.C22_CHARGE [order 1] : after(VPulseW,msec)
          | [VENT_CMP_DETECT]
      DDDR.Pace.PACE_VENT -> DDDR.Pace.C22_CHARGE : after(VPulseW, msec)
      DDDR.Pace.AVDelay_PERIOD -> DDDR.Pace.PACE_VENT [order 2] : after(AVDelay-APulseW,msec)
    state MODULATION [parallel]
      during: increment = double(LRL-MSR)/double(Reaction); decrement = double(LRL - MSR)/double(Recovery);
      Target = double(LRL) - (Activity - ActThresh)/double(17 - Response)*2000;
      settings: executionOrder=2
      state STEPUP
        entry:
        ModRate = ModRate - increment/100;
      state START
        entry:
        ModRate = double(LRL);
      state MAXIMUM
        entry:
        ModRate = double(MSR);
      state STEPDOWN
        entry:
        ModRate = ModRate + decrement/100;
      DDDR.MODULATION.STEPUP -> DDDR.MODULATION.STEPUP [order 2] : after(10,msec)[ModRate > Target]
      DDDR.MODULATION.START -> DDDR.MODULATION.STEPUP : [Target < LRL]
      DDDR.MODULATION.STEPUP -> DDDR.MODULATION.MAXIMUM [order 1] : [ModRate <= MSR]
      DDDR.MODULATION.STEPUP -> DDDR.MODULATION.STEPDOWN [order 3] : after(10,msec)
          | [ModRate <= Target]
      DDDR.MODULATION.STEPDOWN -> DDDR.MODULATION.STEPUP [order 3] : after(10,msec)
          | [ModRate >= Target]
      (default) -> DDDR.MODULATION.START
      DDDR.MODULATION.STEPDOWN -> DDDR.MODULATION.START [order 1] : [ModRate >= LRL]
      DDDR.MODULATION.MAXIMUM -> DDDR.MODULATION.STEPDOWN : [Target > MSR]
      DDDR.MODULATION.STEPDOWN -> DDDR.MODULATION.STEPDOWN [order 2] : after(10, msec)[ModRate < Target]
  note: Mode 9
  note: Mode 10
  note: Mode 11
  note: Mode 12
  (default) -> MODE_SELECTION
  MODE_SELECTION -> VOO [order 2] : [Mode==2]
  MODE_SELECTION -> AOO [order 1] : [Mode==1]
  VOO -> MODE_SELECTION : [Mode~=2]
  AOO -> MODE_SELECTION : [Mode~=1]
  MODE_SELECTION -> AAI [order 3] : [Mode==3]
  MODE_SELECTION -> VVI [order 4] : [Mode==4]
  AAI -> MODE_SELECTION : [Mode~=3]
  VVI -> MODE_SELECTION : [Mode~=4]
  MODE_SELECTION -> AOOR [order 5] : [Mode==5]
  MODE_SELECTION -> VOOR [order 6] : [Mode==6]
  AOOR -> MODE_SELECTION : [Mode~=5]
  VOOR -> MODE_SELECTION : [Mode~=6]
  MODE_SELECTION -> VVIR [order 8] : [Mode==8]
  MODE_SELECTION -> AAIR [order 7] : [Mode==7]
  AAIR -> MODE_SELECTION : [Mode~=7]
  VVIR -> MODE_SELECTION : [Mode~=8]
  MODE_SELECTION -> DOO [order 9] : [Mode==9]
  DOO -> MODE_SELECTION : [Mode~=9]
  MODE_SELECTION -> DOOR [order 10] : [Mode==10]
  DOOR -> MODE_SELECTION : [Mode~=10]
  DDD -> MODE_SELECTION : [Mode~=11]
  MODE_SELECTION -> DDD [order 11] : [Mode==11]
  DDDR -> MODE_SELECTION : [Mode~=12]
  MODE_SELECTION -> DDDR [order 12] : [Mode==12]
  data: LRL input uint16; AAmplitude input uint16; APulseW input uint16; ASensitivity input uint16; ARP input uint16; VAmplitude input uint16; VPulseW input uint16; VSensitivity input uint16; VRP input uint16; Reaction input uint16; ActThresh input double; Response input uint16; PACE_CHARGE_CTRL output uint16; VENT_CMP_REF_PWM output uint16; Z_ATR_CTRL output uint16; PACING_REF_PWM output uint16; ATR_CMP_REF_PWM output uint16; Z_VENT_CTRL output uint16; ATR_PACE_CTRL output uint16; VENT_PACE_CTRL output uint16; PACE_GND_CTRL output uint16; ATR_GND_CTRL output uint16; VENT_GND_CTRL output uint16; Mode input uint16; Recovery input uint16; FRONTEND_CTRL output uint16; RED_LED output uint16; GREEN_LED output uint16; BLUE_LED output uint16; ATR_CMP_DETECT input boolean; VENT_CMP_DETECT input boolean; AVDelay input uint16; Activity input double; ModRate local double; MSR input uint16; Target local double; decrement local double; increment local double
